simulink model "Wall_Model_06Sep18_2016"  (R2018a)
settings: Solver=ode3  StartTime=0.0  StopTime=inf  FixedStep=Ts  RelTol=1e-3  EnableMultiTasking=on
InitFcn:
  | Ts=1;
  | Duration=36000;
  | %% Coefficients of Rs and Cs
  | y1 = 0.5
  | x1 = 0.33;
  | y2 = 0.5;
  | x2 = 0.33;
  | y3 = 1;
  | x3 = 0.33;
  | 
  | T1_initial=28;
  | T2_initial=27;
  | 
  | %% Resistance and Capacitance of Wall
  | Rth = 1/0.8; % Common building brick conductivity = 0.8
  | Cth = 1000; % average thermal capcitance
undefined symbols (not defined in the file or in its folder): x4
libraries: powerlib x66
settings Model: Creator=elekkr  LastModifiedBy=e0154145
settings DataIOCC: LimitDataPoints=on  SaveFormat=Array
settings OptimizationCC: LifeSpan=inf
settings DebuggingCC: UnconnectedInputMsg=none  UnconnectedOutputMsg=none  UnconnectedLineMsg=none  SFUnexpectedBacktrackingDiag=warning  SFNoUnconditionalDefaultTransitionDiag=warning  SFExecutionAtInitializationDiag=none
settings HardwareCC: ProdBitPerPointer=32  ProdBitPerSizeT=32  ProdBitPerPtrDiffT=32  ProdLargestAtomicFloat=None  ProdIntDivRoundTo=Undefined  ProdEndianess=Unspecified  ProdWordSize=32  ProdHWDeviceType=32-bit Generic
settings ModelReferenceCC: PropagateSignalLabelsOutOfModel=off
settings CodeAppCC: StateflowObjectComments=on
settings GRTTargetCC: TargetLangStandard=C89/C90 (ANSI)  GeneratePreprocessorConditionals=Disable all
settings ConfigComp: CovMetricSettings=dw  CovHtmlReporting=on  CovSaveCumulativeToWorkspaceVar=on  CovSaveSingleToWorkspaceVar=on  CovExternalEMLEnable=off
settings SimscapeCC: SimscapeNormalizeSystem=off

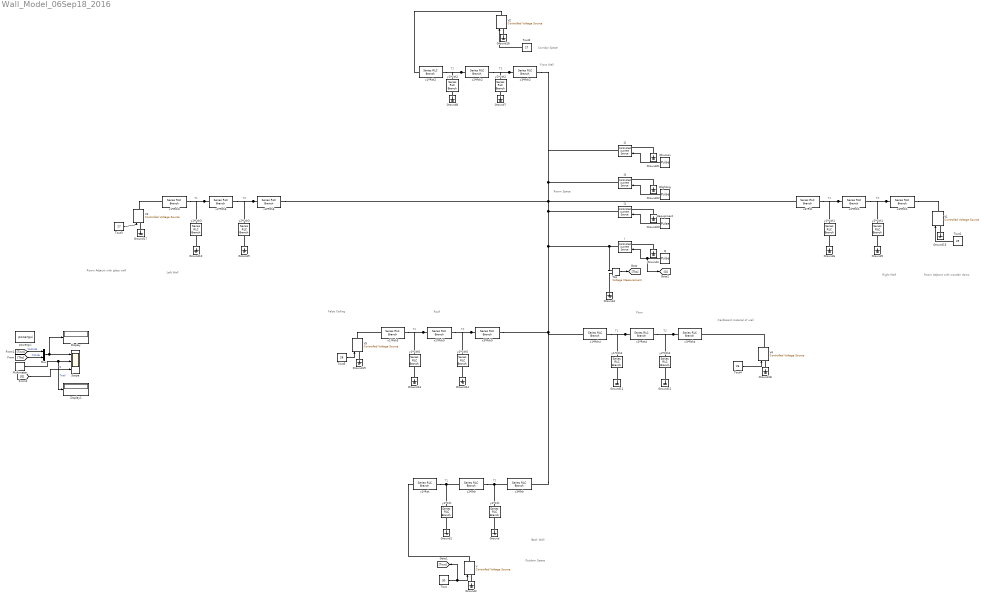
== system Wall_Model_06Sep18_2016 ==
  note: T1
  note: T2
  note: Back Wall
  note: Room Space
  note: Outdoor Space
  note: T1
  note: T2
  note: T1
  note: T2
  note: T1
  note: T2
  note: T2
  note: T1
  note: T1
  note: T2
  note: Right Wall
  note: Front Wall
  note: Left Wall
  note: Floor
  note: Roof
  note: Room Adjacnt with glass wall
  note: Corridpr Space
  note: Room Adjacnt with wooden doors
  note: Cardboard material of wall
  note: False Ceiling
  Display : Display
  Display1 : Display
  Ground{,1..22} (23 alike) : powerlib/Elements/Ground  LConnTagsString=a
  I{,1..3} (4 alike) : powerlib/Electrical Sources/Controlled Current Source  Initialize=on  Source_Type=AC  Amplitude=0  Phase=0  Frequency=0  Measurements=None
  Multimeter : powerlib/Measurements/Multimeter  PhasorSimulation=off  OutputType=Complex  sel=[1 2]  L=12  Gain=[1 1]  yselected={'Ub: y1*Cth','Ub: y2*Cth'};  PSBOutputType=1  PSBequivalent=0  AxesSetting=[0,0.1,-100,100]  Display=0  SavedBlockNames=-11
  Mux : Mux  Inputs=2
  Q : DiscretePulseGenerator  PulseType=Time based  Amplitude=-5  Period=1e5  PulseWidth=50  PhaseDelay=1e4
  Qequipment : DiscretePulseGenerator  PulseType=Time based  Period=1e5  PulseWidth=50  PhaseDelay=1e4
  Qhuman : DiscretePulseGenerator  PulseType=Time based  Amplitude=0.5  Period=1e5  PulseWidth=50  PhaseDelay=1e4
  Qlighting : DiscretePulseGenerator  PulseType=Time based  Amplitude=0.75  Period=1e5  PulseWidth=50  PhaseDelay=1e4
  Scope : Scope  NumInputPorts=3
  Tbs : powerlib/Measurements/Voltage Measurement  PhasorSimulation=off  OutputType=Complex  PSBequivalent=0
  Tout : Constant  Value=30
  Tout1 : Constant  Value=25
  Tout2 : Constant  Value=27
  Tout3 : Constant  Value=27
  Tout4 : Constant  Value=26
  Tout5 : Constant  Value=28
  V{,1..5} (6 alike) : powerlib/Electrical Sources/Controlled Voltage Source  Initialize=on  Source_Type=AC  Amplitude=0  Phase=0  Frequency=0  Measurements=None
  powergui : powerlib/powergui  Priority=1  SimulationMode=Discrete  SampleTime=Ts  frequency=60  Iterations=50  frequencyindice=0  Pbase=100e6  ErrMax=1e-4  UnitsV=kV  UnitsW=MW  buscounter=0  FunctionMessages=off  echomessages=off  EnableUseOfTLC=off  CurrentSourceSwitches=off  DisableSnubberDevices=off  DisableRonSwitches=off  DisableVfSwitches=off  DisplayEquations=off  SolverType=Tustin/Backward Euler (TBE)  Interpol=off  ExternalGateDelay=off  methode=off  Ts=100  x0status=blocks  SPID=off  SwTol=0  HookPort=off  RestoreLinks=warning  ResistiveCurrentMeasurement=off  Frange=[0:2:500]  Ylog=off  Xlog=on  ShowGrid=off  save=off  variable=ZData  structure=0  ZoomFFT=off  StartTime=0.0  cycles=1  DisplayStyle=1  fundamental=60  FreqAxis=off  MaxFrequency=1000  frequencyindicesteady=1  RmsSteady=1  display=off
  x1*Rth{,2..5} (5 alike) : powerlib/Elements/Series RLC Branch  LConnTagsString=__new0  RConnTagsString=__new0  BranchType=R  Resistance=x1*Rth  Inductance=1e-3  SetiL0=off  InitialCurrent=0  Capacitance=1e-6  Setx0=off  InitialVoltage=0  Measurements=None
  x2*Rth{,1..5} (6 alike) : powerlib/Elements/Series RLC Branch  LConnTagsString=__new0  RConnTagsString=__new0  BranchType=R  Resistance=x2*Rth  Inductance=1e-3  SetiL0=off  InitialCurrent=0  Capacitance=1e-6  Setx0=off  InitialVoltage=0  Measurements=None
  x3*Rth{,1..5} (6 alike) : powerlib/Elements/Series RLC Branch  LConnTagsString=__new0  RConnTagsString=__new0  BranchType=R  Resistance=x3*Rth  Inductance=1e-3  SetiL0=off  InitialCurrent=0  Capacitance=1e-6  Setx0=off  InitialVoltage=0  Measurements=None
  x4*Rth : powerlib/Elements/Series RLC Branch  LConnTagsString=__new0  RConnTagsString=__new0  BranchType=R  Resistance=x4*Rth  Inductance=1e-3  SetiL0=off  InitialCurrent=0  Capacitance=1e-6  Setx0=off  InitialVoltage=0  Measurements=None
  y1*Cth{,1..5} (6 alike) : powerlib/Elements/Series RLC Branch  LConnTagsString=__new0  RConnTagsString=__new0  BranchType=C  Resistance=0  Inductance=1e-3  SetiL0=off  InitialCurrent=0  Capacitance=y1*Cth  Setx0=on  InitialVoltage=T1_initial  Measurements=Branch voltage
  y2*Cth{,1..5} (6 alike) : powerlib/Elements/Series RLC Branch  LConnTagsString=__new0  RConnTagsString=__new0  BranchType=C  Resistance=0  Inductance=1e-3  SetiL0=off  InitialCurrent=0  Capacitance=y2*Cth  Setx0=on  InitialVoltage=T2_initial  Measurements=Branch voltage
  wires:
  Q/1 -> [Q], I/1
  Tout/1 -> [Tout], V/1
  Tbs/1 -> [Tbs]
  Mux/1 -> Display/1, Scope/1
  [Tbs] -> Mux/2  "Tinside"
  [Tout] -> Mux/1  "Toutside"
  Multimeter/1 -> Display1/1, Scope/2  "Twall"
  [Q] -> Scope/3  "Q"
  Tout1/1 -> V1/1
  Tout2/1 -> V2/1
  Tout3/1 -> V3/1
  Tout4/1 -> V4/1
  Tout5/1 -> V5/1
  Qequipment/1 -> I1/1
  Qhuman/1 -> I2/1
  Qlighting/1 -> I3/1
  connections:
  x1*Rth/RConn1 -- y1*Cth/LConn1 -- x2*Rth/LConn1
  x2*Rth/RConn1 -- y2*Cth/LConn1 -- x3*Rth/LConn1
  x4*Rth/LConn1 -- I2/RConn1 -- x3*Rth2/RConn1 -- I3/RConn1 -- x3*Rth3/RConn1 -- I1/RConn1 -- Tbs/LConn1 -- I/RConn1 -- x1*Rth4/LConn1 -- x3*Rth/RConn1 -- x3*Rth5/RConn1
  Ground/LConn1 -- y2*Cth/RConn1
  Ground1/LConn1 -- y1*Cth/RConn1
  V/RConn1 -- x1*Rth/LConn1
  Ground2/LConn1 -- V/LConn1
  Ground3/LConn1 -- I/LConn1
  Ground4/LConn1 -- Tbs/LConn2
  x3*Rth1/LConn1 -- x2*Rth1/RConn1 -- y2*Cth1/LConn1
  x2*Rth1/LConn1 -- x4*Rth/RConn1 -- y1*Cth1/LConn1
  Ground5/LConn1 -- y2*Cth1/RConn1
  Ground6/LConn1 -- y1*Cth1/RConn1
  x3*Rth2/LConn1 -- x2*Rth2/RConn1 -- y2*Cth2/LConn1
  x2*Rth2/LConn1 -- x1*Rth2/RConn1 -- y1*Cth2/LConn1
  Ground7/LConn1 -- y2*Cth2/RConn1
  Ground8/LConn1 -- y1*Cth2/RConn1
  x3*Rth3/LConn1 -- x2*Rth3/RConn1 -- y2*Cth3/LConn1
  x2*Rth3/LConn1 -- x1*Rth3/RConn1 -- y1*Cth3/LConn1
  Ground9/LConn1 -- y2*Cth3/RConn1
  Ground10/LConn1 -- y1*Cth3/RConn1
  x2*Rth4/LConn1 -- x1*Rth4/RConn1 -- y1*Cth4/LConn1
  x3*Rth4/LConn1 -- x2*Rth4/RConn1 -- y2*Cth4/LConn1
  Ground11/LConn1 -- y1*Cth4/RConn1
  Ground12/LConn1 -- y2*Cth4/RConn1
  x3*Rth5/LConn1 -- x2*Rth5/RConn1 -- y2*Cth5/LConn1
  x2*Rth5/LConn1 -- x1*Rth5/RConn1 -- y1*Cth5/LConn1
  Ground13/LConn1 -- y1*Cth5/RConn1
  Ground14/LConn1 -- y2*Cth5/RConn1
  Ground15/LConn1 -- V1/LConn1
  x1*Rth2/LConn1 -- V2/RConn1
  Ground16/LConn1 -- V2/LConn1
  x1*Rth3/LConn1 -- V3/RConn1
  Ground17/LConn1 -- V3/LConn1
  Ground18/LConn1 -- V4/LConn1
  x1*Rth5/LConn1 -- V5/RConn1
  Ground19/LConn1 -- V5/LConn1
  Ground20/LConn1 -- I1/LConn1
  Ground21/LConn1 -- I2/LConn1
  Ground22/LConn1 -- I3/LConn1
  x3*Rth1/RConn1 -- V1/RConn1
  V4/RConn1 -- x3*Rth4/RConn1
